simulink model "EPA_Walker"  (R2018a)
settings: Solver=FixedStepDiscrete  StartTime=0.0  StopTime=inf  FixedStep=0.001  RelTol=1e-3  EnableMultiTasking=on
model workspace (MAT data in the model file):
  k_p_pam = Simulink.Parameter
  k_p_pam.DataType = 'auto'
  k_p_pam.Dimensions = [0 0]
undefined symbols (not defined in the file or in its folder): bits_current, bits_GRF, bits_Kd, bits_Kp, bits_position, bits_velocity, deadzone_in_TIB, deadzone_out_TIB, GRF_MAX, GRF_MIN, k_p_TIB, KD_MAX, KD_MIN, KP_MAX, KP_MIN, P_MAX, P_MIN, PressureFilter_CutOffFreq, PressureFilter_Gain, ReadingVoltage, T_MAX, T_MIN, V_MAX, V_MIN, voltageBias_GAS, voltageBias_GL, voltageBias_HAM, voltageBias_IL, voltageBias_POP, voltageBias_RF, voltageBias_SOL, voltageBias_TIB, voltageBias_VAS, voltageMultiplier_GAS, voltageMultiplier_GL, voltageMultiplier_HAM, voltageMultiplier_IL, voltageMultiplier_POP, voltageMultiplier_RF, voltageMultiplier_SOL, voltageMultiplier_TIB, voltageMultiplier_VAS, VoltageResolution
libraries: xpcethercatlib x139, simulink x19, peGeneralControl x18, slrtlib x9
(part 1 of 5)
settings Model: xpc_rtwmakecfg_data=_xpcethercatlib_  ModifiedComment=marcm -- Wed Oct 11 08:58:17 2023 -- Version 1.614  SimulationMode=external  Creator=marcm  LastModifiedBy=marcm
settings Model: ModifiedHistory=|
  | marcm -- Wed Oct 11 08:58:17 2023 -- Version 1.614
  | 
  | marcm -- Wed Oct 11 06:47:10 2023 -- Version 1.613
  | 
  | marcm -- Wed Oct 11 06:45:06 2023 -- Version 1.612
  | 
  | marcm -- Wed Oct 11 06:36:01 2023 -- Version 1.611
  | 
  | marcm -- Wed Oct 11 06:35:34 2023 -- Version 1.610
  | 
  | marcm -- Wed Oct 11 06:16:40 2023 -- Version 1.609
  | 
  | marcm -- Wed Oct 11 06:03:46 2023 -- Version 1.608
  | 
  | marcm -- Wed Oct 11 06:00:18 2023 -- Version 1.607
  | 
  | marcm -- Wed Oct 11 05:59:50 2023 -- Version 1.606
  | 
  | marcm -- Wed Oct 11 05:58:49 2023 -- Version 1.605
  | 
  | marcm -- Wed Oct 11 05:45:44 2023 -- Version 1.604
  | 
  | marcm -- Tue Oct 10 10:18:13 2023 -- Version 1.603
  | 
  | marcm -- Tue Oct 10 10:17:09 2023 -- Version 1.602
  | 
  | marcm -- Tue Oct 10 10:16:55 2023 -- Version 1.601
  | 
  | marcm -- Tue Oct 10 10:16:41 2023 -- Version 1.600
  | 
  | marcm -- Tue Oct 10 09:54:37 2023 -- Version 1.599
  | 
  | marcm -- Tue Oct 10 09:52:33 2023 -- Version 1.598
  | 
  | marcm -- Tue Oct 10 09:52:19 2023 -- Version 1.597
  | 
  | marcm -- Tue Oct 10 09:49:28 2023 -- Version 1.596
  | 
  | marcm -- Tue Oct 10 09:46:34 2023 -- Version 1.595
  | 
  | marcm -- Tue Oct 10 09:40:05 2023 -- Version 1.594
  | 
  | marcm -- Tue Oct 10 09:39:53 2023 -- Version 1.593
  | 
  | marcm -- Tue Oct 10 09:25:46 2023 -- Version 1.592
  | 
  | marcm -- Tue Oct 10 09:23:35 2023 -- Version 1.591
  | 
  | marcm -- Tue Oct 10 09:23:25 2023 -- Version 1.590
  | 
  | marcm -- Tue Oct 10 09:22:37 2023 -- Version 1.589
  | 
  | marcm -- Tue Oct 10 09:21:28 2023 -- Version 1.588
  | 
  | marcm -- Tue Oct 10 09:21:20 2023 -- Version 1.587
  | 
  | marcm -- Tue Oct 10 09:20:22 2023 -- Version 1.586
  | 
  | marcm -- Tue Oct 10 09:19:32 2023 -- Version 1.585
  | 
  | marcm -- Tue Oct 10 09:13:59 2023 -- Version 1.584
  | 
  | marcm -- Tue Oct 10 09:13:07 2023 -- Version 1.583
  | 
  | marcm -- Tue Oct 10 09:10:28 2023 -- Version 1.582
  | 
  | marcm -- Tue Oct 10 09:08:57 2023 -- Version 1.581
  | 
  | marcm -- Tue Oct 10 09:04:23 2023 -- Version 1.580
  | 
  | marcm -- Tue Oct 10 09:04:07 2023 -- Version 1.579
  | 
  | marcm -- Tue Oct 10 09:04:01 2023 -- Version 1.578
  | 
  | marcm -- Tue Oct 10 09:02:40 2023 -- Version 1.577
  | 
  | marcm -- Tue Oct 10 09:02:15 2023 -- Version 1.576
  | 
  | marcm -- Tue Oct 10 09:01:35 2023 -- Version 1.575
  | 
  | marcm -- Tue Oct 10 08:50:29 2023 -- Version 1.574
  | 
  | marcm -- Tue Oct 10 08:46:42 2023 -- Version 1.573
  | 
  | marcm -- Tue Oct 10 08:46:16 2023 -- Version 1.572
  | 
  | marcm -- Tue Oct 10 08:41:23 2023 -- Version 1.571
  | 
  | marcm -- Tue Oct 10 08:40:45 2023 -- Version 1.569
  | 
  | marcm -- Tue Oct 10 08:40:45 2023 -- Version 1.569
  | 
  | marcm -- Tue Oct 10 08:40:18 2023 -- Version 1.568
  | 
  | marcm -- Tue Oct 10 08:39:51 2023 -- Version 1.567
  | 
  | marcm -- Tue Oct 10 08:39:28 2023 -- Version 1.566
  | 
  | marcm -- Tue Oct 10 08:36:32 2023 -- Version 1.564
  | 
  | marcm -- Tue Oct 10 08:36:32 2023 -- Version 1.564
  | 
  | marcm -- Tue Oct 10 08:34:28 2023 -- Version 1.562
  | 
  | marcm -- Tue Oct 10 08:34:28 2023 -- Version 1.562
  | 
  | marcm -- Tue Oct 10 08:30:52 2023 -- Version 1.561
  | 
  | marcm -- Tue Oct 10 07:37:16 2023 -- Version 1.560
  | 
  | marcm -- Tue Oct 10 07:37:06 2023 -- Version 1.559
  | 
  | marcm -- Tue Oct 10 07:36:57 2023 -- Version 1.558
  | 
  | marcm -- Tue Oct 10 07:36:51 2023 -- Version 1.557
  | 
  | marcm -- Tue Oct 10 07:30:00 2023 -- Version 1.556
  | 
  | marcm -- Tue Oct 10 07:27:11 2023 -- Version 1.555
  | 
  | marcm -- Tue Oct 10 07:22:37 2023 -- Version 1.554
  | 
  | marcm -- Tue Oct 10 07:13:40 2023 -- Version 1.553
  | 
  | marcm -- Tue Oct 10 07:09:54 2023 -- Version 1.552
  | 
  | marcm -- Tue Oct 10 07:09:31 2023 -- Version 1.551
  | 
  | marcm -- Tue Oct 10 07:08:00 2023 -- Version 1.550
  | 
  | marcm -- Tue Oct 10 07:04:41 2023 -- Version 1.549
  | 
  | marcm -- Tue Oct 10 07:01:53 2023 -- Version 1.548
  | 
  | marcm -- Tue Oct 10 06:59:36 2023 -- Version 1.547
  | 
  | marcm -- Fri Oct 06 03:41:09 2023 -- Version 1.546
settings SolverCC: ConcurrentTasks=on  AutoInsertRateTranBlk=on
settings DataIOCC: SaveFormat=StructureWithTime
settings OptimizationCC: BlockReduction=off  OptimizeBlockIOStorage=off  BufferReuse=off  GlobalBufferReuse=off  ExpressionFolding=off  LocalBlockOutputs=off  OptimizeDataStoreBuffers=off  BusAssignmentInplaceUpdate=off
settings HardwareCC: ProdBitPerPointer=32  ProdBitPerSizeT=32  ProdBitPerPtrDiffT=32  ProdLargestAtomicFloat=None  ProdWordSize=32  ProdLongLongMode=on  ProdHWDeviceType=Generic->32-bit x86 compatible
settings RTWCC: SystemTargetFile=slrt.tlc  TemplateMakefile=slrt_default_tmf  Description=Simulink Real-Time  CodeExecutionProfiling=on  RTWCompilerOptimization=on
settings CodeAppCC: StateflowObjectComments=on
settings SimulinkRealTimeCC: SupportVariableSizeSignals=on  xPCConcurrentTasks=on

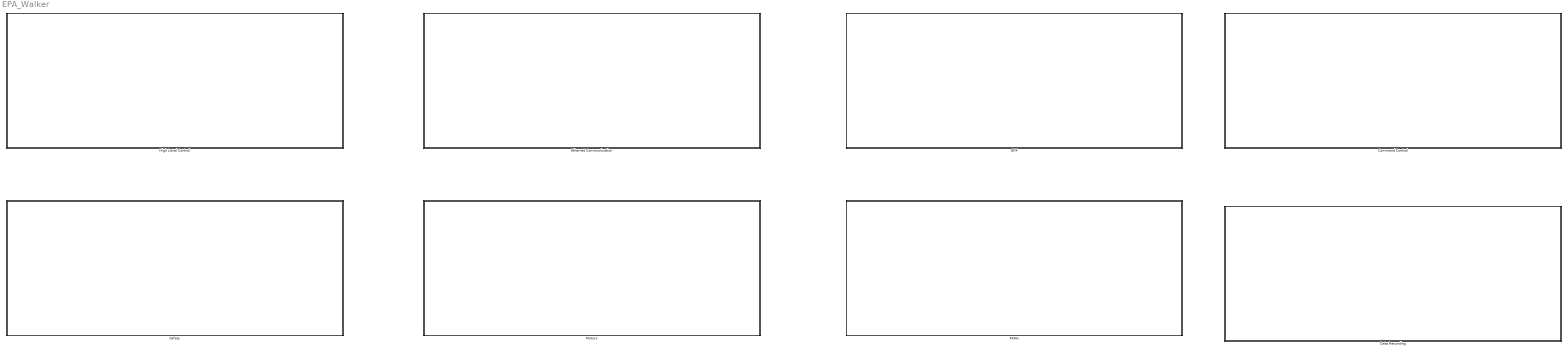
== system EPA_Walker ==
  Command Control : Subsystem
  Data Recording : Subsystem
  Ethernet Communication : Subsystem
  GRF : Subsystem
  High Level Control : Subsystem
  Motors : Subsystem
  PAMs : Subsystem
  "Safety " : Subsystem

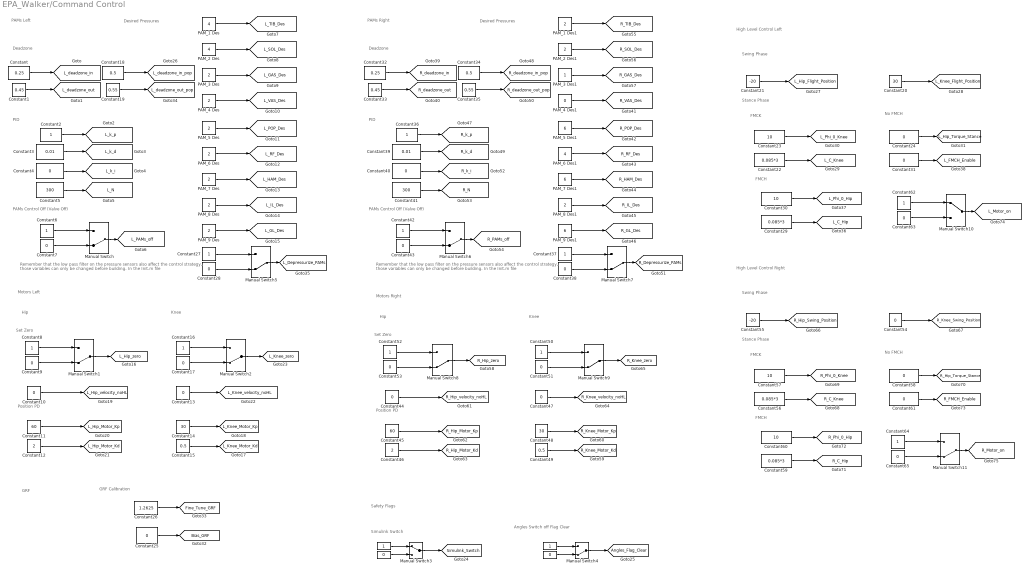
== system EPA_Walker/Command Control ==
  note: PID
  note: PAMs Left
  note: Deadzone
  note: PAMs Control Off (Valve Off)
  note: Desired Pressures
  note: Motors Left
  note: Remember that the low pass filter on the pressure sensors also affect the control strategy, those variables can only be changed before building. In the Init.m file
  note: Hip
  note: Knee
  note: Safety Flags
  note: Simulink Switch
  note: Angles Switch off Flag Clear
  note: GRF
  note: High Level Control Left
  note: Swing Phase
  note: Stance Phase
  note: FMCK
  note: Position PD
  note: Set Zero
  note: GRF Calibration
  note: No FMCH
  note: FMCH
  note: Deadzone
  note: PAMs Control Off (Valve Off)
  note: Desired Pressures
  note: PAMs Right
  note: Remember that the low pass filter on the pressure sensors also affect the control strategy, those variables can only be changed before building. In the Init.m file
  note: PID
  note: Position PD
  note: Motors Right
  note: Hip
  note: Knee
  note: Set Zero
  note: High Level Control Right
  note: FMCK
  note: Stance Phase
  note: No FMCH
  note: Swing Phase
  note: FMCH
  " " : Constant
  "   " : Constant  Value=0
  "    " : Constant  Value=0
  "               " : Constant
  Constant : Constant  Value=0.25
  Constant1 : Constant  Value=0.45
  Constant{4,7,9..10,13,17,24..25,28,31,38,40,43..44,47,51,53..54,58,61,63,65} (22 alike) : Constant  Value=0
  Constant11 : Constant  Value=60
  Constant12 : Constant  Value=2
  Constant14 : Constant  Value=30
  Constant{15,18,34,49} (4 alike) : Constant  Value=0.5
  Constant{2,6,8,16,27,36..37,42,50,52,62,64} (12 alike) : Constant
  Constant19 : Constant  Value=0.55
  Constant20 : Constant  Value=30
  Constant21 : Constant  Value=-20
  Constant{22,29,56,59} (4 alike) : Constant  Value=0.085*3
  Constant{23,30,57,60} (4 alike) : Constant  Value=10
  Constant26 : Constant  Value=1.2625
  Constant3 : Constant  Value=0.01
  Constant32 : Constant  Value=0.25
  Constant33 : Constant  Value=0.45
  Constant35 : Constant  Value=0.55
  Constant39 : Constant  Value=0.01
  Constant41 : Constant  Value=300
  Constant45 : Constant  Value=60
  Constant46 : Constant  Value=2
  Constant48 : Constant  Value=30
  Constant5 : Constant  Value=300
  Constant55 : Constant  Value=-20
  Manual Switch{,1..2,4..9,11} (10 alike) : ManualSwitch  CurrentSetting=0
  Manual Switch10 : ManualSwitch
  Manual Switch3 : ManualSwitch
  PAM_1 Des : Constant  Value=4
  PAM_1 Des1 : Constant  Value=2
  PAM_2 Des : Constant  Value=4
  PAM_2 Des1 : Constant  Value=2
  PAM_3 Des : Constant  Value=2
  PAM_3 Des1 : Constant
  PAM_4 Des : Constant  Value=2
  PAM_4 Des1 : Constant  Value=0
  PAM_5 Des : Constant  Value=2
  PAM_5 Des1 : Constant  Value=6
  PAM_6 Des : Constant  Value=2
  PAM_6 Des1 : Constant  Value=4
  PAM_7 Des : Constant  Value=2
  PAM_7 Des1 : Constant  Value=6
  PAM_8 Des : Constant  Value=2
  PAM_8 Des1 : Constant  Value=2
  PAM_9 Des : Constant  Value=2
  PAM_9 Des1 : Constant  Value=6
  tag scope: Angles_Flag_Clear=global, Bias_GRF=global, Fine_Tune_GRF=global, L_C_Hip=global, L_C_Knee=global, L_Depressurize_PAMs=global, L_FMCH_Enable=global, L_GAS_Des=global, L_GL_Des=global, L_HAM_Des=global, L_Hip_Flight_Position=global, L_Hip_Motor_Kd=global, L_Hip_Motor_Kp=global, L_Hip_Torque_Stance=global, L_Hip_velocity_noHL=global, L_Hip_zero=global, L_IL_Des=global, L_Knee_Flight_Position=global, L_Knee_Motor_Kd=global, L_Knee_Motor_Kp=global, L_Knee_velocity_noHL=global, L_Knee_zero=global, L_Motor_on=global, L_N=global, L_PAMs_off=global, L_POP_Des=global, L_Phi_0_Hip=global, L_Phi_0_Knee=global, L_RF_Des=global, L_SOL_Des=global, L_TIB_Des=global, L_VAS_Des=global, L_deadzone_in=global, L_deadzone_in_pop=global, L_deadzone_out=global, L_deadzone_out_pop=global, L_k_d=global, L_k_i=global, L_k_p=global, R_C_Hip=global, R_C_Knee=global, R_Depressurize_PAMs=global, R_FMCH_Enable=global, R_GAS_Des=global, R_GL_Des=global, R_HAM_Des=global, R_Hip_Motor_Kd=global, R_Hip_Motor_Kp=global, R_Hip_Swing_Position=global, R_Hip_Torque_Stance=global, R_Hip_velocity_noHL=global, R_Hip_zero=global, R_IL_Des=global, R_Knee_Motor_Kd=global, R_Knee_Motor_Kp=global, R_Knee_Swing_Position=global, R_Knee_velocity_noHL=global, R_Knee_zero=global, R_Motor_on=global, R_N=global, R_PAMs_off=global, R_POP_Des=global, R_Phi_0_Hip=global, R_Phi_0_Knee=global, R_RF_Des=global, R_SOL_Des=global, R_TIB_Des=global, R_VAS_Des=global, R_deadzone_in=global, R_deadzone_in_pop=global, R_deadzone_out=global, R_deadzone_out_pop=global, R_k_d=global, R_k_i=global, R_k_p=global, Simulink_Switch=global
  wires:
  Constant5/1 -> [L_N]
  Constant4/1 -> [L_k_i]
  Constant6/1 -> Manual Switch/1
  Manual Switch/1 -> [L_PAMs_off]
  Constant1/1 -> [L_deadzone_out]
  Constant7/1 -> Manual Switch/2
  Constant2/1 -> [L_k_p]
  Constant/1 -> [L_deadzone_in]
  Constant3/1 -> [L_k_d]
  PAM_1 Des/1 -> [L_TIB_Des]
  PAM_2 Des/1 -> [L_SOL_Des]
  PAM_3 Des/1 -> [L_GAS_Des]
  PAM_4 Des/1 -> [L_VAS_Des]
  PAM_5 Des/1 -> [L_POP_Des]
  PAM_6 Des/1 -> [L_RF_Des]
  PAM_7 Des/1 -> [L_HAM_Des]
  PAM_8 Des/1 -> [L_IL_Des]
  PAM_9 Des/1 -> [L_GL_Des]
  Constant8/1 -> Manual Switch1/1
  Constant9/1 -> Manual Switch1/2
  Manual Switch1/1 -> [L_Hip_zero]
  Constant10/1 -> [L_Hip_velocity_noHL]
  Constant11/1 -> [L_Hip_Motor_Kp]
  Constant12/1 -> [L_Hip_Motor_Kd]
  Constant13/1 -> [L_Knee_velocity_noHL]
  Constant14/1 -> [L_Knee_Motor_Kp]
  Constant15/1 -> [L_Knee_Motor_Kd]
  Manual Switch2/1 -> [L_Knee_zero]
  Constant17/1 -> Manual Switch2/2
  Constant16/1 -> Manual Switch2/1
  " "/1 -> Manual Switch3/1
  "    "/1 -> Manual Switch3/2
  Manual Switch3/1 -> [Simulink_Switch]
  Manual Switch4/1 -> [Angles_Flag_Clear]
  "               "/1 -> Manual Switch4/1
  "   "/1 -> Manual Switch4/2
  Constant21/1 -> [L_Hip_Flight_Position]
  Constant20/1 -> [L_Knee_Flight_Position]
  Constant23/1 -> [L_Phi_0_Knee]
  Constant22/1 -> [L_C_Knee]
  Constant24/1 -> [L_Hip_Torque_Stance]
  Constant25/1 -> [Bias_GRF]
  Constant26/1 -> [Fine_Tune_GRF]
  Constant18/1 -> [L_deadzone_in_pop]
  Constant19/1 -> [L_deadzone_out_pop]
  Constant27/1 -> Manual Switch5/1
  Constant28/1 -> Manual Switch5/2
  Manual Switch5/1 -> [L_Depressurize_PAMs]
  Constant30/1 -> [L_Phi_0_Hip]
  Constant29/1 -> [L_C_Hip]
  Constant31/1 -> [L_FMCH_Enable]
  Manual Switch6/1 -> [R_PAMs_off]
  PAM_6 Des1/1 -> [R_RF_Des]
  PAM_4 Des1/1 -> [R_VAS_Des]
  PAM_3 Des1/1 -> [R_GAS_Des]
  PAM_2 Des1/1 -> [R_SOL_Des]
  Constant33/1 -> [R_deadzone_out]
  Constant43/1 -> Manual Switch6/2
  PAM_1 Des1/1 -> [R_TIB_Des]
  Constant32/1 -> [R_deadzone_in]
  Constant37/1 -> Manual Switch7/1
  Constant41/1 -> [R_N]
  Constant35/1 -> [R_deadzone_out_pop]
  PAM_5 Des1/1 -> [R_POP_Des]
  PAM_7 Des1/1 -> [R_HAM_Des]
  Constant39/1 -> [R_k_d]
  Manual Switch7/1 -> [R_Depressurize_PAMs]
  PAM_9 Des1/1 -> [R_GL_Des]
  Constant42/1 -> Manual Switch6/1
  Constant34/1 -> [R_deadzone_in_pop]
  Constant38/1 -> Manual Switch7/2
  PAM_8 Des1/1 -> [R_IL_Des]
  Constant40/1 -> [R_k_i]
  Constant36/1 -> [R_k_p]
  Constant45/1 -> [R_Hip_Motor_Kp]
  Constant52/1 -> Manual Switch8/1
  Constant51/1 -> Manual Switch9/2
  Manual Switch9/1 -> [R_Knee_zero]
  Constant49/1 -> [R_Knee_Motor_Kd]
  Constant53/1 -> Manual Switch8/2
  Manual Switch8/1 -> [R_Hip_zero]
  Constant47/1 -> [R_Knee_velocity_noHL]
  Constant50/1 -> Manual Switch9/1
  Constant48/1 -> [R_Knee_Motor_Kp]
  Constant44/1 -> [R_Hip_velocity_noHL]
  Constant46/1 -> [R_Hip_Motor_Kd]
  Constant54/1 -> [R_Knee_Swing_Position]
  Constant57/1 -> [R_Phi_0_Knee]
  Constant59/1 -> [R_C_Hip]
  Constant61/1 -> [R_FMCH_Enable]
  Constant58/1 -> [R_Hip_Torque_Stance]
  Constant56/1 -> [R_C_Knee]
  Constant55/1 -> [R_Hip_Swing_Position]
  Constant60/1 -> [R_Phi_0_Hip]
  Constant62/1 -> Manual Switch10/1
  Constant63/1 -> Manual Switch10/2
  Manual Switch10/1 -> [L_Motor_on]
  Constant64/1 -> Manual Switch11/1
  Constant65/1 -> Manual Switch11/2
  Manual Switch11/1 -> [R_Motor_on]

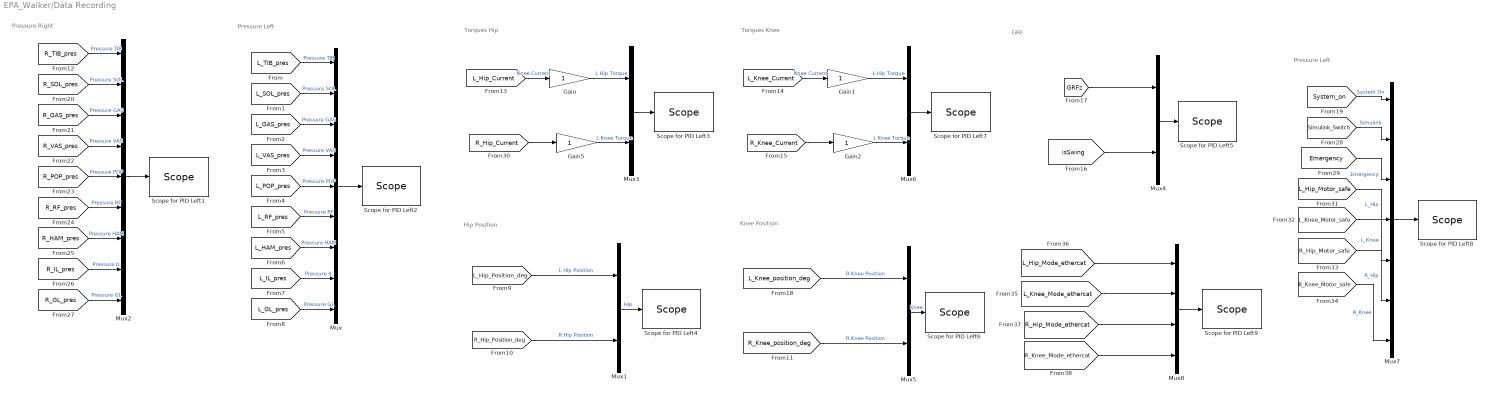
== system EPA_Walker/Data Recording ==
  note: GRF
  note: Hip Position
  note: Knee Position
  note: Torques Hip
  note: Pressure Left
  note: Pressure Right
  note: Torques Knee
  note: Pressure Left
  Gain{,1..2,5} (4 alike) : Gain
  Mux : Mux  Inputs=9
  Mux{1,3..6} (5 alike) : Mux  Inputs=2
  Mux2 : Mux  Inputs=9
  Mux7 : Mux  Inputs=7
  Mux8 : Mux
  Scope for PID Left1 : slrtlib/Displays and Logging/Scope   scopeno=7  scopetype=Target  autostart=on  viewmode=Numerical  formatstr='%15.6f'  grid=on  ylimits=[0, 0]  nosamples=1000  noprepostsamples=0  interleave=1  triggermode=FreeRun  triggersignal=1  trigsignalfromport=off  triggerlevel=0.0  triggerslope=Either  triggerscope=1  triggersample=0  filename=data.dat  mode=Lazy  writesize=512  autorestart=off  dynamicfilemode=off  maxwritefilesize=512*1024^2
  Scope for PID Left2 : slrtlib/Displays and Logging/Scope   scopeno=8  scopetype=Target  autostart=on  viewmode=Numerical  formatstr='%15.6f'  grid=on  ylimits=[0, 0]  nosamples=1000  noprepostsamples=0  interleave=1  triggermode=FreeRun  triggersignal=1  trigsignalfromport=off  triggerlevel=0.0  triggerslope=Either  triggerscope=1  triggersample=0  filename=data.dat  mode=Lazy  writesize=512  autorestart=off  dynamicfilemode=off  maxwritefilesize=512*1024^2
  Scope for PID Left3 : slrtlib/Displays and Logging/Scope   scopeno=3  scopetype=Target  autostart=on  viewmode=Graphical sliding  formatstr='%15.6f'  grid=on  ylimits=[0, 0]  nosamples=1000  noprepostsamples=0  interleave=1  triggermode=FreeRun  triggersignal=1  trigsignalfromport=off  triggerlevel=0.0  triggerslope=Either  triggerscope=1  triggersample=0  filename=data.dat  mode=Lazy  writesize=512  autorestart=off  dynamicfilemode=off  maxwritefilesize=512*1024^2
  Scope for PID Left4 : slrtlib/Displays and Logging/Scope   scopeno=2  scopetype=Target  autostart=on  viewmode=Graphical sliding  formatstr='%15.6f'  grid=on  ylimits=[-60, 60]  nosamples=1000  noprepostsamples=0  interleave=1  triggermode=FreeRun  triggersignal=1  trigsignalfromport=off  triggerlevel=0.0  triggerslope=Either  triggerscope=1  triggersample=0  filename=data.dat  mode=Lazy  writesize=512  autorestart=off  dynamicfilemode=off  maxwritefilesize=512*1024^2
  Scope for PID Left5 : slrtlib/Displays and Logging/Scope   scopeno=4  scopetype=Target  autostart=on  viewmode=Graphical sliding  formatstr='%15.6f'  grid=on  ylimits=[0, 0]  nosamples=1000  noprepostsamples=0  interleave=1  triggermode=FreeRun  triggersignal=1  trigsignalfromport=off  triggerlevel=0.0  triggerslope=Either  triggerscope=1  triggersample=0  filename=data.dat  mode=Lazy  writesize=512  autorestart=off  dynamicfilemode=off  maxwritefilesize=512*1024^2
  Scope for PID Left6 : slrtlib/Displays and Logging/Scope   scopeno=5  scopetype=Target  autostart=on  viewmode=Graphical sliding  formatstr='%15.6f'  grid=on  ylimits=[-60, 60]  nosamples=1000  noprepostsamples=0  interleave=1  triggermode=FreeRun  triggersignal=1  trigsignalfromport=off  triggerlevel=0.0  triggerslope=Either  triggerscope=1  triggersample=0  filename=data.dat  mode=Lazy  writesize=512  autorestart=off  dynamicfilemode=off  maxwritefilesize=512*1024^2
  Scope for PID Left7 : slrtlib/Displays and Logging/Scope   scopeno=6  scopetype=Target  autostart=on  viewmode=Graphical sliding  formatstr='%15.6f'  grid=on  ylimits=[0, 0]  nosamples=1000  noprepostsamples=0  interleave=1  triggermode=FreeRun  triggersignal=1  trigsignalfromport=off  triggerlevel=0.0  triggerslope=Either  triggerscope=1  triggersample=0  filename=data.dat  mode=Lazy  writesize=512  autorestart=off  dynamicfilemode=off  maxwritefilesize=512*1024^2
  Scope for PID Left8 : slrtlib/Displays and Logging/Scope   scopeno=1  scopetype=Target  autostart=on  viewmode=Numerical  formatstr='%15.6f'  grid=on  ylimits=[0, 0]  nosamples=1000  noprepostsamples=0  interleave=1  triggermode=FreeRun  triggersignal=1  trigsignalfromport=off  triggerlevel=0.0  triggerslope=Either  triggerscope=1  triggersample=0  filename=data.dat  mode=Lazy  writesize=512  autorestart=off  dynamicfilemode=off  maxwritefilesize=512*1024^2
  Scope for PID Left9 : slrtlib/Displays and Logging/Scope   scopeno=9  scopetype=Target  autostart=on  viewmode=Numerical  formatstr='%15.6f'  grid=on  ylimits=[0, 0]  nosamples=1000  noprepostsamples=0  interleave=1  triggermode=FreeRun  triggersignal=1  trigsignalfromport=off  triggerlevel=0.0  triggerslope=Either  triggerscope=1  triggersample=0  filename=data.dat  mode=Lazy  writesize=512  autorestart=off  dynamicfilemode=off  maxwritefilesize=512*1024^2
  wires:
  [L_POP_pres] -> Mux/5  "Pressure POP"
  [L_TIB_pres] -> Mux/1  "Pressure TIB"
  Mux/1 -> Scope for PID Left2/1
  [L_RF_pres] -> Mux/6  "Pressure RF"
  [L_GAS_pres] -> Mux/3  "Pressure GAS"
  [L_HAM_pres] -> Mux/7  "Pressure HAM"
  [L_GL_pres] -> Mux/9  "Pressure GL"
  [L_VAS_pres] -> Mux/4  "Pressure VAS"
  [L_SOL_pres] -> Mux/2  "Pressure SOL"
  [L_IL_pres] -> Mux/8  "Pressure IL"
  [L_Hip_Current] -> Gain/1  "Knee Current"
  Mux3/1 -> Scope for PID Left3/1
  [R_Hip_Position_deg] -> Mux1/2  "R Hip Position"
  Gain/1 -> Mux3/1  "L Hip Torque"
  Gain5/1 -> Mux3/2  "L Knee Torque"
  Mux1/1 -> Scope for PID Left4/1  "Hip"
  [R_Hip_Current] -> Gain5/1
  [L_Hip_Position_deg] -> Mux1/1  "L Hip Position"
  [GRFz] -> Mux4/1
  Mux4/1 -> Scope for PID Left5/1
  [isSwing] -> Mux4/2
  [R_Knee_position_deg] -> Mux5/2  "R Knee Position"
  [L_Knee_position_deg] -> Mux5/1  "R Knee Position"
  Mux5/1 -> Scope for PID Left6/1  "Knee"
  [R_IL_pres] -> Mux2/8  "Pressure IL"
  [R_GL_pres] -> Mux2/9  "Pressure GL"
  [R_RF_pres] -> Mux2/6  "Pressure RF"
  [R_HAM_pres] -> Mux2/7  "Pressure HAM"
  [R_TIB_pres] -> Mux2/1  "Pressure TIB"
  [R_VAS_pres] -> Mux2/4  "Pressure VAS"
  Mux2/1 -> Scope for PID Left1/1
  [R_POP_pres] -> Mux2/5  "Pressure POP"
  [R_SOL_pres] -> Mux2/2  "Pressure SOL"
  [R_GAS_pres] -> Mux2/3  "Pressure GAS"
  Mux6/1 -> Scope for PID Left7/1
  [L_Knee_Current] -> Gain1/1  "Knee Current"
  [R_Knee_Current] -> Gain2/1
  Gain1/1 -> Mux6/1  "L Hip Torque"
  Gain2/1 -> Mux6/2  "L Knee Torque"
  [R_Hip_Motor_safe] -> Mux7/6  "R_Hip"
  [R_Knee_Motor_safe] -> Mux7/7  "R_Knee"
  [System_on] -> Mux7/1  "System On"
  [L_Hip_Motor_safe] -> Mux7/4  "L_Hip"
  Mux7/1 -> Scope for PID Left8/1
  [L_Knee_Motor_safe] -> Mux7/5  "L_Knee"
  [Simulink_Switch] -> Mux7/2  "Simulink"
  [Emergency] -> Mux7/3  "Emergency"
  [L_Hip_Mode_ethercat] -> Mux8/1
  [L_Knee_Mode_ethercat] -> Mux8/2
  Mux8/1 -> Scope for PID Left9/1
  [R_Hip_Mode_ethercat] -> Mux8/3
  [R_Knee_Mode_ethercat] -> Mux8/4

== system EPA_Walker/Ethernet Communication ==
  "EtherCAT Get Notifications " : xpcethercatlib/EtherCAT Get Notifications   device_id=0  sample_time=.001
      settings: SourceProductName=Simulink Real-Time  SourceProductBaseCode=XP
  "EtherCAT Init " : xpcethercatlib/EtherCAT Init   Priority=0  config_file=C:\Users\marcm\PhD\EPA-Walker\RealTime Code\XML_files\EPA_Walker_v0.xml  device_id=0  pci_bus=3  pci_slot=0  pci_function=0  dctuning=0  enaDebug=off  enaDC=on  errLink=off  masterDbg=off  stateChgDbg=off  baseClock=off  masterCfg=off  logFile='c:\dbglog.txt'  sample_time=0.001000  DCMode=0
      settings: SourceProductName=Simulink Real-Time  SourceProductBaseCode=XP
  Inputs : Subsystem
  Outputs : Subsystem
  Terminator : Terminator
  Terminator1 : Terminator
  wires:
  "EtherCAT Get Notifications "/1 -> Terminator1/1
  "EtherCAT Init "/1 -> Terminator/1

== system EPA_Walker/GRF ==
  note: GRF Meassures
  2D-Vector : Subsystem
  GRFx : Subsystem
  GRFy : Subsystem
  GRFz : Subsystem

== system EPA_Walker/High Level Control ==
  Delay : Delay  DelayLength=1
  HL Left : Subsystem
  HL Right : Subsystem
  Walking Phase Detection : MATLAB Function  TreatAsAtomicUnit=on
  tag scope: isSwing=global
  wires:
  Walking Phase Detection/1(isSwing) -> Delay/1, [isSwing], HL Left/1(isSwing), HL Right/1(isSwing)  "isSwing"
  [GRFz] -> Walking Phase Detection/1(GRFz)
  Delay/1 -> Walking Phase Detection/2(previous_isSwing)

== system EPA_Walker/Motors ==
  Motor Left : Subsystem
  Motor Right : Subsystem

== system EPA_Walker/PAMs ==
  PAMs Left : Subsystem
  PAMs Right : Subsystem

== system EPA_Walker/Safety  ==
  AND1 : Logic  Inputs=3  IconShape=distinctive  AllPortsSameDT=off  OutDataTypeStr=boolean
  Constant : Constant
  Data Type Conversion3 : DataTypeConversion  OutDataTypeStr=double
  Delay : Delay  DelayLength=1  InitialCondition=0  ExternalReset=Either
      settings: InputPortMap=u0,r5
  Delay1 : Delay  DelayLength=1  InitialCondition=0  ExternalReset=Either
      settings: InputPortMap=u0,r5
  MATLAB Function : MATLAB Function  TreatAsAtomicUnit=on
  MATLAB Function1 : MATLAB Function  TreatAsAtomicUnit=on
  Manual Switch : ManualSwitch
  System On : Subsystem
  tag scope: L_Hip_Motor_safe=global, L_Knee_Motor_safe=global, R_Hip_Motor_safe=global, R_Knee_Motor_safe=global, System_on=global
  wires:
  System On/1(System On) -> AND1/1  "System On"
  [Simulink_Switch] -> System On/1("Simulink Switch ")  "Simulink Switch"
  [L_Hip_Position_deg] -> MATLAB Function/1(Hip_Position)
  MATLAB Function/3(Motors_safe) -> AND1/2  "Motors_safe"
  MATLAB Function/1(Hip_motor_safe) -> [L_Hip_Motor_safe]  "Hip_motor_safe"
  MATLAB Function/2(Knee_motor_safe) -> [L_Knee_Motor_safe]  "Knee_motor_safe"
  AND1/1 -> Data Type Conversion3/1
  MATLAB Function/4(flag) -> Delay/1
  Delay/1 -> MATLAB Function/3(flag_1)
  [Angles_Flag_Clear] -> Delay/2
  [L_Knee_position_deg] -> MATLAB Function/2(Knee_Position)
  MATLAB Function1/4(flag) -> Delay1/1
  MATLAB Function1/3(Motors_safe) -> AND1/3  "Motors_safe"
  Delay1/1 -> MATLAB Function1/3(flag_1)
  [R_Hip_Position_deg] -> MATLAB Function1/1(Hip_Position)
  [R_Knee_position_deg] -> MATLAB Function1/2(Knee_Position)
  [Angles_Flag_Clear] -> Delay1/2
  MATLAB Function1/2(Knee_motor_safe) -> [R_Knee_Motor_safe]  "Knee_motor_safe"
  MATLAB Function1/1(Hip_motor_safe) -> [R_Hip_Motor_safe]  "Hip_motor_safe"
  Data Type Conversion3/1 -> Manual Switch/1
  Manual Switch/1 -> [System_on]
  Constant/1 -> Manual Switch/2

== system EPA_Walker/Ethernet Communication/Inputs ==
  GRF Slave : Subsystem
  Motor Left : Subsystem
  Motor Right : Subsystem
  PAMs Left : Subsystem
  PAMs Right : Subsystem

== system EPA_Walker/Ethernet Communication/Outputs ==
  GRF Slave : Subsystem
  Motor Left : Subsystem
  Motor Right : Subsystem
  PAMs Left : Subsystem
  PAMs Right : Subsystem

== system EPA_Walker/GRF/2D-Vector ==
  Asin : Trigonometry  Operator=asin
  Divide : Product  Inputs=*/
  Sqrt : Sqrt  SaturateOnIntegerOverflow=on
  Square : Math  Operator=square  SaturateOnIntegerOverflow=on
  Square1 : Math  Operator=square  SaturateOnIntegerOverflow=on
  Sum : Sum  Inputs=+|+
  tag scope: GRF_VectAng=global, GRF_VectMag=global
  wires:
  [GRFy] -> Square/1
  [GRFz] -> Square1/1
  Square/1 -> Sum/1
  Square1/1 -> Divide/1, Sum/2
  Sum/1 -> Sqrt/1
  Sqrt/1 -> Divide/2, [GRF_VectMag]  "GRF Vector"
  Divide/1 -> Asin/1
  Asin/1 -> [GRF_VectAng]  "GRF Angle"

== system EPA_Walker/GRF/GRFx ==
  note: GRF Low Pass Filter
  Constant17 : Constant  Value=0
  Constant18 : Constant
  Filter : DiscreteFilter  Numerator="[0.0036    0.0072    0.0036]"  Denominator="[1.0000   -1.8227    0.8372]"  ExternalReset=Either
      settings: InputPortMap=u0,r7
  Gain27 : Gain  Gain=100
  Sum3 : Sum  Inputs=|+-
  tag scope: GRFx=global
  wires:
  Gain27/1 -> Sum3/1
  Sum3/1 -> Filter/1
  Filter/1 -> [GRFx]  "GRF z"
  Constant17/1 -> Sum3/2
  Constant18/1 -> Filter/2
  [GRFx_Volts] -> Gain27/1

== system EPA_Walker/GRF/GRFy ==
  note: GRF Low Pass Filter
  Constant17 : Constant  Value=0
  Constant18 : Constant
  Filter : DiscreteFilter  Numerator="[0.0036    0.0072    0.0036]"  Denominator="[1.0000   -1.8227    0.8372]"  ExternalReset=Either
      settings: InputPortMap=u0,r7
  Gain27 : Gain  Gain=200
  Sum3 : Sum  Inputs=|+-
  tag scope: GRFy=global
  wires:
  Gain27/1 -> Sum3/1
  Sum3/1 -> Filter/1
  Filter/1 -> [GRFy]  "GRF y"
  Constant17/1 -> Sum3/2
  Constant18/1 -> Filter/2
  [GRFy_Volts] -> Gain27/1

== system EPA_Walker/GRF/GRFz ==
  note: GRF Low Pass Filter
  Constant18 : Constant
  Filter : DiscreteFilter  Numerator="[0.0036    0.0072    0.0036]"  Denominator="[1.0000   -1.8227    0.8372]"  ExternalReset=Either
      settings: InputPortMap=u0,r7
  Gain27 : Gain  Gain=300
  Multiply : Product
  Sum3 : Sum  Inputs=|+-
  tag scope: GRFz=global
  wires:
  Constant18/1 -> Filter/2
  [Bias_GRF] -> Sum3/2
  Sum3/1 -> Filter/1
  [GRFz_Volts] -> Gain27/1
  Filter/1 -> [GRFz]  "GRF z"
  Gain27/1 -> Multiply/1
  Multiply/1 -> Sum3/1
  [Fine_Tune_GRF] -> Multiply/2

== system EPA_Walker/High Level Control/HL Left ==
  isSwing : Inport
  Logical Operator : Logic  Operator=NOT  AllPortsSameDT=off  OutDataTypeStr=boolean
  Motor Modes : MATLAB Function  TreatAsAtomicUnit=on
  Stance phase : Subsystem
  Swing phase : Subsystem
  tag scope: L_Hip_mode=global, L_Hip_position_HL=global, L_Hip_torque_HL=global, L_Knee_mode=global, L_Knee_position_HL=global, L_Knee_torque_HL=global
  wires:
  isSwing/1 -> Logical Operator/1, Motor Modes/1(isSwing), Swing phase/Enable
  Logical Operator/1 -> Stance phase/Enable
  [L_Phi_0_Hip] -> Stance phase/8(Phi_0_Hip)
  Stance phase/1(Hip_torque_HL) -> [L_Hip_torque_HL]
  Stance phase/2(Knee_torque_HL) -> [L_Knee_torque_HL]
  [L_Hip_Position_deg] -> Stance phase/6(Hip)
  Motor Modes/2(Knee_mode) -> [L_Knee_mode]
  Swing phase/1(Hip) -> [L_Hip_position_HL]
  [L_C_Hip] -> Stance phase/7(C_Hip)
  Motor Modes/1(Hip_mode) -> [L_Hip_mode]
  [L_Hip_Flight_Position] -> Swing phase/1(Hip_Position_Des_swing)
  [L_Knee_Flight_Position] -> Swing phase/2(Knee_Position_Des_swing)
  [L_Phi_0_Knee] -> Stance phase/4(Phi_0_Knee)
  [L_Hip_Torque_Stance] -> Stance phase/5(Hip_Torque_Stance)
  [GRFz] -> Stance phase/1("GRFz ")
  [L_Knee_position_deg] -> Stance phase/2(Knee)
  [L_FMCH_Enable] -> Stance phase/9(FMCH Enable)
  [L_C_Knee] -> Stance phase/3(C_Knee)
  Swing phase/2(Knee) -> [L_Knee_position_HL]

== system EPA_Walker/High Level Control/HL Right ==
  isSwing : Inport
  Logical Operator : Logic  Operator=NOT  AllPortsSameDT=off  OutDataTypeStr=boolean
  Motor Modes : MATLAB Function  TreatAsAtomicUnit=on
  Stance phase : Subsystem
  Swing phase : Subsystem
  tag scope: R_Hip_mode=global, R_Hip_position_HL=global, R_Hip_torque_HL=global, R_Knee_mode=global, R_Knee_position_HL=global, R_Knee_torque_HL=global
  wires:
  isSwing/1 -> Logical Operator/1, Motor Modes/1(isSwing), Swing phase/Enable
  Logical Operator/1 -> Stance phase/Enable
  [R_Phi_0_Hip] -> Stance phase/8(Phi_0_Hip)
  Stance phase/1(Hip_torque_HL) -> [R_Hip_torque_HL]
  Stance phase/2(Knee_torque_HL) -> [R_Knee_torque_HL]
  [R_Hip_Position_deg] -> Stance phase/6(Hip)
  Motor Modes/2(Knee_mode) -> [R_Knee_mode]
  Swing phase/1(Hip) -> [R_Hip_position_HL]
  [R_C_Hip] -> Stance phase/7(C_Hip)
  Motor Modes/1(Hip_mode) -> [R_Hip_mode]
  [R_Hip_Swing_Position] -> Swing phase/1(Hip_Position_Des_flight)
  [R_Knee_Swing_Position] -> Swing phase/2(Knee_Position_Des_flight)
  [R_Phi_0_Knee] -> Stance phase/4(Phi_0_Knee)
  [R_Hip_Torque_Stance] -> Stance phase/5(Hip_Torque_Stance)
  [GRFz] -> Stance phase/1("GRFz ")
  [R_Knee_position_deg] -> Stance phase/2(Knee)
  [R_FMCH_Enable] -> Stance phase/9(FMCH Enable)
  [R_C_Knee] -> Stance phase/3(C_Knee)
  Swing phase/2(Knee) -> [R_Knee_position_HL]

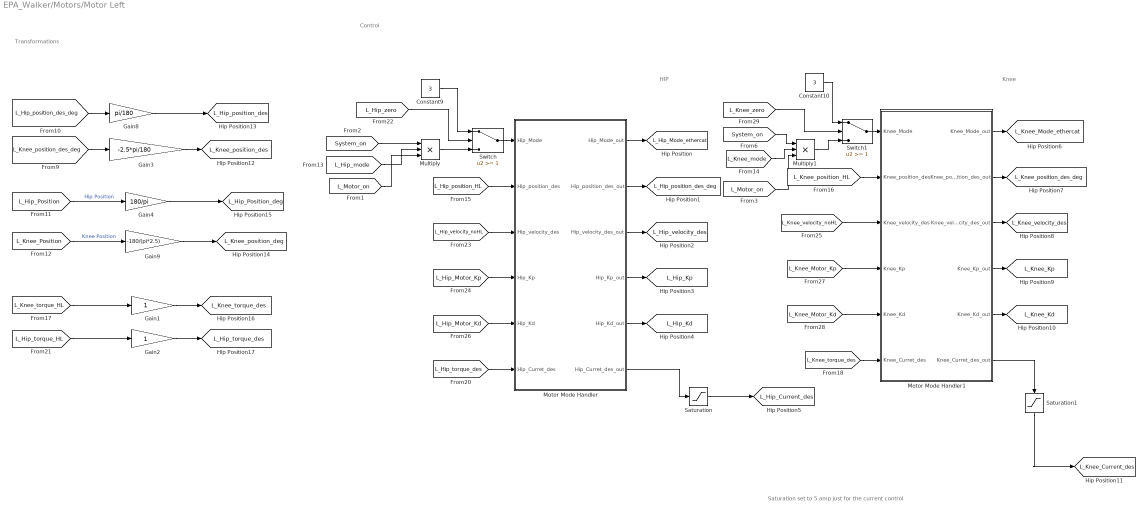
== system EPA_Walker/Motors/Motor Left ==
  note: Saturation set to 5 amp just for the current control
  note: HIP
  note: Knee
  note: Control
  note: Transformations
  Constant10 : Constant  Value=3
  Constant9 : Constant  Value=3
  Gain1 : Gain
  Gain2 : Gain
  Gain3 : Gain  Gain=-2.5*pi/180
  Gain4 : Gain  Gain=180/pi
  Gain8 : Gain  Gain=pi/180
  Gain9 : Gain  Gain=-180/(pi*2.5)
  Motor Mode Handler : MATLAB Function  TreatAsAtomicUnit=on
  Motor Mode Handler1 : MATLAB Function  TreatAsAtomicUnit=on
  Multiply : Product  Inputs=3
  Multiply1 : Product  Inputs=3
  Saturation : Saturate  UpperLimit=5  LowerLimit=-5
  Saturation1 : Saturate  UpperLimit=5  LowerLimit=-5
  Switch : Switch  Threshold=1
  Switch1 : Switch  Threshold=1
  tag scope: L_Hip_Current_des=global, L_Hip_Kd=global, L_Hip_Kp=global, L_Hip_Mode_ethercat=global, L_Hip_Position_deg=global, L_Hip_position_des=global, L_Hip_position_des_deg=global, L_Hip_torque_des=global, L_Hip_velocity_des=global, L_Knee_Current_des=global, L_Knee_Kd=global, L_Knee_Kp=global, L_Knee_Mode_ethercat=global, L_Knee_position_deg=global, L_Knee_position_des=global, L_Knee_position_des_deg=global, L_Knee_torque_des=global, L_Knee_velocity_des=global
  wires:
  [L_Hip_position_des_deg] -> Gain8/1
  [System_on] -> Multiply/1
  Motor Mode Handler/5(Hip_Kd_out) -> [L_Hip_Kd]
  [L_Hip_torque_des] -> Motor Mode Handler/6(Hip_Curret_des)
  [L_Hip_Motor_Kp] -> Motor Mode Handler/4(Hip_Kp)
  [L_Hip_velocity_noHL] -> Motor Mode Handler/3(Hip_velocity_des)
  [L_Hip_Position] -> Gain4/1  "Hip Position"
  [L_Hip_position_HL] -> Motor Mode Handler/2(Hip_position_des)
  Motor Mode Handler1/5(Knee_Kd_out) -> [L_Knee_Kd]
  Motor Mode Handler1/2(Knee_position_des_out) -> [L_Knee_position_des_deg]
  Motor Mode Handler1/3(Knee_velocity_des_out) -> [L_Knee_velocity_des]
  [L_Hip_torque_HL] -> Gain2/1
  Constant9/1 -> Switch/1
  [System_on] -> Multiply1/1
  [L_Knee_torque_HL] -> Gain1/1
  Motor Mode Handler1/4(Knee_Kp_out) -> [L_Knee_Kp]
  Constant10/1 -> Switch1/1
  [L_Hip_mode] -> Multiply/2
  Motor Mode Handler1/1(Knee_Mode_out) -> [L_Knee_Mode_ethercat]
  [L_Knee_Position] -> Gain9/1  "Knee Position"
  [L_Knee_Motor_Kp] -> Motor Mode Handler1/4(Knee_Kp)
  [L_Knee_torque_des] -> Motor Mode Handler1/6(Knee_Curret_des)
  [L_Knee_zero] -> Switch1/2
  [L_Knee_Motor_Kd] -> Motor Mode Handler1/5(Knee_Kd)
  Gain8/1 -> [L_Hip_position_des]
  Motor Mode Handler/4(Hip_Kp_out) -> [L_Hip_Kp]
  Motor Mode Handler/3(Hip_velocity_des_out) -> [L_Hip_velocity_des]
  [L_Knee_mode] -> Multiply1/2
  Switch/1 -> Motor Mode Handler/1(Hip_Mode)
  [L_Hip_zero] -> Switch/2
  Gain2/1 -> [L_Hip_torque_des]
  [L_Knee_velocity_noHL] -> Motor Mode Handler1/3(Knee_velocity_des)
  Gain1/1 -> [L_Knee_torque_des]
  Multiply1/1 -> Switch1/3
  Motor Mode Handler1/6(Knee_Curret_des_out) -> Saturation1/1
  Gain9/1 -> [L_Knee_position_deg]
  Gain4/1 -> [L_Hip_Position_deg]
  [L_Knee_position_HL] -> Motor Mode Handler1/2(Knee_position_des)
  [L_Knee_position_des_deg] -> Gain3/1
  Motor Mode Handler/1(Hip_Mode_out) -> [L_Hip_Mode_ethercat]
  Gain3/1 -> [L_Knee_position_des]
  Motor Mode Handler/6(Hip_Curret_des_out) -> Saturation/1
  Saturation/1 -> [L_Hip_Current_des]
  Motor Mode Handler/2(Hip_position_des_out) -> [L_Hip_position_des_deg]
  Saturation1/1 -> [L_Knee_Current_des]
  Multiply/1 -> Switch/3
  [L_Hip_Motor_Kd] -> Motor Mode Handler/5(Hip_Kd)
  Switch1/1 -> Motor Mode Handler1/1(Knee_Mode)
  [L_Motor_on] -> Multiply/3
  [L_Motor_on] -> Multiply1/3

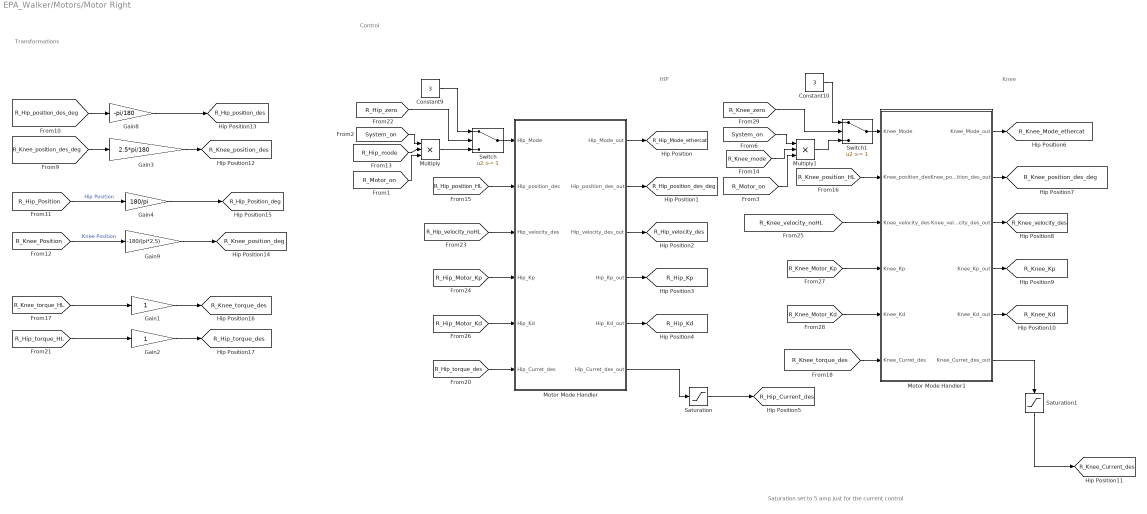
== system EPA_Walker/Motors/Motor Right ==
  note: HIP
  note: Knee
  note: Transformations
  note: Control
  note: Saturation set to 5 amp just for the current control
  Constant10 : Constant  Value=3
  Constant9 : Constant  Value=3
  Gain1 : Gain
  Gain2 : Gain
  Gain3 : Gain  Gain=2.5*pi/180
  Gain4 : Gain  Gain=180/pi
  Gain8 : Gain  Gain=-pi/180
  Gain9 : Gain  Gain=-180/(pi*2.5)
  Motor Mode Handler : MATLAB Function  TreatAsAtomicUnit=on
  Motor Mode Handler1 : MATLAB Function  TreatAsAtomicUnit=on
  Multiply : Product  Inputs=3
  Multiply1 : Product  Inputs=3
  Saturation : Saturate  UpperLimit=5  LowerLimit=-5
  Saturation1 : Saturate  UpperLimit=5  LowerLimit=-5
  Switch : Switch  Threshold=1
  Switch1 : Switch  Threshold=1
  tag scope: R_Hip_Current_des=global, R_Hip_Kd=global, R_Hip_Kp=global, R_Hip_Mode_ethercat=global, R_Hip_Position_deg=global, R_Hip_position_des=global, R_Hip_position_des_deg=global, R_Hip_torque_des=global, R_Hip_velocity_des=global, R_Knee_Current_des=global, R_Knee_Kd=global, R_Knee_Kp=global, R_Knee_Mode_ethercat=global, R_Knee_position_deg=global, R_Knee_position_des=global, R_Knee_position_des_deg=global, R_Knee_torque_des=global, R_Knee_velocity_des=global
  wires:
  Motor Mode Handler1/3(Knee_velocity_des_out) -> [R_Knee_velocity_des]
  Motor Mode Handler1/2(Knee_position_des_out) -> [R_Knee_position_des_deg]
  [R_Hip_velocity_noHL] -> Motor Mode Handler/3(Hip_velocity_des)
  [R_Hip_mode] -> Multiply/2
  Motor Mode Handler1/5(Knee_Kd_out) -> [R_Knee_Kd]
  [R_Hip_torque_des] -> Motor Mode Handler/6(Hip_Curret_des)
  [R_Hip_Position] -> Gain4/1  "Hip Position"
  [R_Hip_position_HL] -> Motor Mode Handler/2(Hip_position_des)
  [R_Knee_Motor_Kd] -> Motor Mode Handler1/5(Knee_Kd)
  [R_Knee_mode] -> Multiply1/2
  [R_Knee_Position] -> Gain9/1  "Knee Position"
  [R_Hip_zero] -> Switch/2
  [R_Hip_Motor_Kp] -> Motor Mode Handler/4(Hip_Kp)
  Motor Mode Handler1/4(Knee_Kp_out) -> [R_Knee_Kp]
  Saturation1/1 -> [R_Knee_Current_des]
  Motor Mode Handler/4(Hip_Kp_out) -> [R_Hip_Kp]
  Switch/1 -> Motor Mode Handler/1(Hip_Mode)
  Gain8/1 -> [R_Hip_position_des]
  Constant10/1 -> Switch1/1
  [R_Knee_position_HL] -> Motor Mode Handler1/2(Knee_position_des)
  Motor Mode Handler/6(Hip_Curret_des_out) -> Saturation/1
  Motor Mode Handler1/1(Knee_Mode_out) -> [R_Knee_Mode_ethercat]
  [R_Knee_velocity_noHL] -> Motor Mode Handler1/3(Knee_velocity_des)
  [R_Hip_torque_HL] -> Gain2/1
  Motor Mode Handler/2(Hip_position_des_out) -> [R_Hip_position_des_deg]
  Motor Mode Handler/3(Hip_velocity_des_out) -> [R_Hip_velocity_des]
  Gain1/1 -> [R_Knee_torque_des]
  [R_Knee_torque_des] -> Motor Mode Handler1/6(Knee_Curret_des)
  Motor Mode Handler/5(Hip_Kd_out) -> [R_Hip_Kd]
  Multiply/1 -> Switch/3
  Gain4/1 -> [R_Hip_Position_deg]
  Multiply1/1 -> Switch1/3
  [R_Knee_zero] -> Switch1/2
  [System_on] -> Multiply/1
  Gain2/1 -> [R_Hip_torque_des]
  [R_Knee_Motor_Kp] -> Motor Mode Handler1/4(Knee_Kp)
  Switch1/1 -> Motor Mode Handler1/1(Knee_Mode)
  [R_Hip_Motor_Kd] -> Motor Mode Handler/5(Hip_Kd)
  Saturation/1 -> [R_Hip_Current_des]
  Motor Mode Handler/1(Hip_Mode_out) -> [R_Hip_Mode_ethercat]
  [R_Knee_position_des_deg] -> Gain3/1
  Motor Mode Handler1/6(Knee_Curret_des_out) -> Saturation1/1
  Gain3/1 -> [R_Knee_position_des]
  Gain9/1 -> [R_Knee_position_deg]
  [R_Knee_torque_HL] -> Gain1/1
  [System_on] -> Multiply1/1
  Constant9/1 -> Switch/1
  [R_Hip_position_des_deg] -> Gain8/1
  [R_Motor_on] -> Multiply/3
  [R_Motor_on] -> Multiply1/3

== system EPA_Walker/PAMs/PAMs Left ==
  GAS : Subsystem
  GL : Subsystem
  HAM : Subsystem
  IL : Subsystem
  POP : Subsystem
  RF : Subsystem
  SOL : Subsystem
  TIB : Subsystem
  VAS : Subsystem
  wires:
  [L_SOL_Des] -> SOL/1(Pressure Des)
  [L_VAS_Des] -> VAS/1(Pressure Des)
  [L_TIB_Des] -> TIB/1(Pressure Des)
  [L_GAS_Des] -> GAS/1(Pressure Des)
  [L_IL_Des] -> IL/1(Pressure Des)
  [L_GL_Des] -> GL/1(Pressure Des)
  [L_HAM_Des] -> HAM/1(Pressure Des)
  [L_RF_Des] -> RF/1(Pressure Des)
  [L_POP_Des] -> POP/1(Pressure Des)

== system EPA_Walker/PAMs/PAMs Right ==
  GAS : Subsystem
  GL : Subsystem
  HAM : Subsystem
  IL : Subsystem
  POP : Subsystem
  RF : Subsystem
  SOL : Subsystem
  TIB : Subsystem
  VAS : Subsystem
  wires:
  [R_SOL_Des] -> SOL/1(Pressure Des)
  [R_VAS_Des] -> VAS/1(Pressure Des)
  [R_TIB_Des] -> TIB/1(Pressure Des)
  [R_GAS_Des] -> GAS/1(Pressure Des)
  [R_IL_Des] -> IL/1(Pressure Des)
  [R_GL_Des] -> GL/1(Pressure Des)
  [R_HAM_Des] -> HAM/1(Pressure Des)
  [R_RF_Des] -> RF/1(Pressure Des)
  [R_POP_Des] -> POP/1(Pressure Des)

== system EPA_Walker/Safety /System On ==
  "Simulink Switch " : Inport
  Clock2 : Clock
  Compare To Constant : simulink/Logic and Bit Operations/Compare To Constant  relop=>=  const=10  OutDataTypeStr=boolean
  Data Type Conversion3 : DataTypeConversion  OutDataTypeStr=double
  Emergency Switch : MATLAB Function  TreatAsAtomicUnit=on
  Logical Operator : Logic  Inputs=3  AllPortsSameDT=off  OutDataTypeStr=boolean
  System On : Outport
  tag scope: Emergency=global
  wires:
  Emergency Switch/1(y) -> [Emergency], Logical Operator/3
  [Emergency_Switch] -> Emergency Switch/1(Emergency_switch)
  "Simulink Switch "/1 -> Logical Operator/2
  Clock2/1 -> Compare To Constant/1
  Compare To Constant/1 -> Logical Operator/1
  Logical Operator/1 -> Data Type Conversion3/1
  Data Type Conversion3/1 -> System On/1

== system EPA_Walker/Ethernet Communication/Inputs/GRF Slave ==
  note: Emergency Switch
  note: GRF
  Data Type Conversion3 : DataTypeConversion
  EtherCAT PDO Receive1 : xpcethercatlib/EtherCAT PDO Receive  Priority=2  sig_name=GRF.Inputs.Byte13  sig_offset=104  sig_type=uint8  type_size=8  sig_dim=1  device_id=0  sample_time=0.001000
      settings: SourceProductName=Simulink Real-Time  SourceProductBaseCode=XP
  EtherCAT PDO Receive2 : xpcethercatlib/EtherCAT PDO Receive  Priority=2  sig_name=GRF.Inputs.Byte14  sig_offset=112  sig_type=uint8  type_size=8  sig_dim=1  device_id=0  sample_time=0.001000
      settings: SourceProductName=Simulink Real-Time  SourceProductBaseCode=XP
  "GRFx " : Subsystem
  "GRFy " : Subsystem
  "GRFz " : Subsystem
  Gain24 : Gain  Gain=256
  Sum5 : Sum
  tag scope: Emergency_Switch=global
  wires:
  Data Type Conversion3/1 -> [Emergency_Switch]
  Gain24/1 -> Sum5/1
  EtherCAT PDO Receive2/1 -> Sum5/2
  Sum5/1 -> Data Type Conversion3/1
  EtherCAT PDO Receive1/1 -> Gain24/1

== system EPA_Walker/Ethernet Communication/Inputs/Motor Left ==
  note: Hip
  note: Knee
  Byte Splitting Hip : MATLAB Function  TreatAsAtomicUnit=on
  Byte Splitting Knee : MATLAB Function  TreatAsAtomicUnit=on
  Data Type Conversion{1..6} (6 alike) : DataTypeConversion
  EtherCAT PDO Receive : xpcethercatlib/EtherCAT PDO Receive  Priority=2  sig_name=Motors_L.Inputs.Byte0  sig_offset=768  sig_type=uint8  type_size=8  sig_dim=1  device_id=0  sample_time=0.001000
      settings: SourceProductName=Simulink Real-Time  SourceProductBaseCode=XP
  EtherCAT PDO Receive1 : xpcethercatlib/EtherCAT PDO Receive  Priority=2  sig_name=Motors_L.Inputs.Byte1  sig_offset=776  sig_type=uint8  type_size=8  sig_dim=1  device_id=0  sample_time=0.001000
      settings: SourceProductName=Simulink Real-Time  SourceProductBaseCode=XP
  EtherCAT PDO Receive2 : xpcethercatlib/EtherCAT PDO Receive  Priority=2  sig_name=Motors_L.Inputs.Byte5  sig_offset=808  sig_type=uint8  type_size=8  sig_dim=1  device_id=0  sample_time=0.001000
      settings: SourceProductName=Simulink Real-Time  SourceProductBaseCode=XP
  EtherCAT PDO Receive3 : xpcethercatlib/EtherCAT PDO Receive  Priority=2  sig_name=Motors_L.Inputs.Byte6  sig_offset=816  sig_type=uint8  type_size=8  sig_dim=1  device_id=0  sample_time=0.001000
      settings: SourceProductName=Simulink Real-Time  SourceProductBaseCode=XP
  EtherCAT PDO Receive4 : xpcethercatlib/EtherCAT PDO Receive  Priority=2  sig_name=Motors_L.Inputs.Byte2  sig_offset=784  sig_type=uint8  type_size=8  sig_dim=1  device_id=0  sample_time=0.001000
      settings: SourceProductName=Simulink Real-Time  SourceProductBaseCode=XP
  EtherCAT PDO Receive5 : xpcethercatlib/EtherCAT PDO Receive  Priority=2  sig_name=Motors_L.Inputs.Byte3  sig_offset=792  sig_type=uint8  type_size=8  sig_dim=1  device_id=0  sample_time=0.001000
      settings: SourceProductName=Simulink Real-Time  SourceProductBaseCode=XP
  EtherCAT PDO Receive6 : xpcethercatlib/EtherCAT PDO Receive  Priority=2  sig_name=Motors_L.Inputs.Byte4  sig_offset=800  sig_type=uint8  type_size=8  sig_dim=1  device_id=0  sample_time=0.001000
      settings: SourceProductName=Simulink Real-Time  SourceProductBaseCode=XP
  EtherCAT PDO Receive7 : xpcethercatlib/EtherCAT PDO Receive  Priority=2  sig_name=Motors_L.Inputs.Byte7  sig_offset=824  sig_type=uint8  type_size=8  sig_dim=1  device_id=0  sample_time=0.001000
      settings: SourceProductName=Simulink Real-Time  SourceProductBaseCode=XP
  EtherCAT PDO Receive8 : xpcethercatlib/EtherCAT PDO Receive  Priority=2  sig_name=Motors_L.Inputs.Byte8  sig_offset=832  sig_type=uint8  type_size=8  sig_dim=1  device_id=0  sample_time=0.001000
      settings: SourceProductName=Simulink Real-Time  SourceProductBaseCode=XP
  EtherCAT PDO Receive9 : xpcethercatlib/EtherCAT PDO Receive  Priority=2  sig_name=Motors_L.Inputs.Byte9  sig_offset=840  sig_type=uint8  type_size=8  sig_dim=1  device_id=0  sample_time=0.001000
      settings: SourceProductName=Simulink Real-Time  SourceProductBaseCode=XP
  Gain{,1,4..5} (4 alike) : Gain  Gain=256
  Gain2 : Gain  Gain=16
  Gain3 : Gain  Gain=16
  Hip Current Transformation : MATLAB Function  TreatAsAtomicUnit=on
  Hip Position Transformation : MATLAB Function  TreatAsAtomicUnit=on
  Hip Velocity Transformation : MATLAB Function  TreatAsAtomicUnit=on
  Knee Current Tranformation : MATLAB Function  TreatAsAtomicUnit=on
  Knee Position Transformation1 : MATLAB Function  TreatAsAtomicUnit=on
  Knee Velocity Transformation1 : MATLAB Function  TreatAsAtomicUnit=on
  Sum{1..6} (6 alike) : Sum
  tag scope: L_Hip_Current=global, L_Hip_Position=global, L_Hip_Velocity=global, L_Knee_Current=global, L_Knee_Position=global, L_Knee_Velocity=global
  wires:
  EtherCAT PDO Receive/1 -> Gain/1
  Sum2/1 -> Data Type Conversion3/1
  Data Type Conversion3/1 -> Hip Position Transformation/1(x_int)
  Gain/1 -> Sum2/1
  EtherCAT PDO Receive1/1 -> Sum2/2
  EtherCAT PDO Receive3/1 -> Sum1/2
  Gain1/1 -> Sum1/1
  Data Type Conversion1/1 -> Knee Position Transformation1/1(x_int)
  EtherCAT PDO Receive2/1 -> Gain1/1
  Sum1/1 -> Data Type Conversion1/1
  EtherCAT PDO Receive5/1 -> Byte Splitting Knee/1(byte)
  EtherCAT PDO Receive4/1 -> Gain2/1
  Gain2/1 -> Sum3/1
  Byte Splitting Knee/1(Vel_low) -> Sum3/2
  EtherCAT PDO Receive6/1 -> Sum4/2
  Data Type Conversion2/1 -> Hip Velocity Transformation/1(x_int)
  Sum3/1 -> Data Type Conversion2/1
  Data Type Conversion4/1 -> Hip Current Transformation/1(x_int)
  Sum4/1 -> Data Type Conversion4/1
  EtherCAT PDO Receive7/1 -> Gain3/1
  Sum5/1 -> Data Type Conversion5/1
  Gain3/1 -> Sum5/1
  EtherCAT PDO Receive9/1 -> Sum6/2
  EtherCAT PDO Receive8/1 -> Byte Splitting Hip/1(byte)
  Byte Splitting Hip/2(Curr_h) -> Gain5/1
  Sum6/1 -> Data Type Conversion6/1
  Byte Splitting Hip/1(Vel_low) -> Sum5/2
  Hip Position Transformation/1(Hip_position) -> [L_Hip_Position]
  Hip Velocity Transformation/1(Hip_velocity) -> [L_Hip_Velocity]
  Hip Current Transformation/1(Hip_current) -> [L_Hip_Current]
  Knee Position Transformation1/1(Knee_position) -> [L_Knee_Position]
  Knee Velocity Transformation1/1(Knee_velocity) -> [L_Knee_Velocity]
  Data Type Conversion5/1 -> Knee Velocity Transformation1/1(x_int)
  Knee Current Tranformation/1(Knee_current) -> [L_Knee_Current]
  Data Type Conversion6/1 -> Knee Current Tranformation/1(x_int)
  Gain4/1 -> Sum4/1
  Byte Splitting Knee/2(Curr_h) -> Gain4/1
  Gain5/1 -> Sum6/1
